simulink model "controller_AWBT"  (R2015a)
settings: Solver=ode5  StartTime=0.0  StopTime=9  FixedStep=1e-4  MaxStep=1e-3  RelTol=1e-3
values from neighbouring files (symbols this model uses):
  Ap = A    [main_matlab_observer.m]    (also in plant.mat = [-1.63570125246 -486.357845111 0 0 486.287213279 -1.89932026)
  Bp = B    [main_matlab_observer.m]    (also in plant.mat = [-8.88712865174  3.42023387272; 4.6056577442  -2.14780344563)
  Cp = C    [main_matlab_observer.m]    (also in plant.mat = [0.096809951598  0.0841099123333  0.0902904274622  -0.004558)
  Hp = E    [main_matlab_observer.m]    (also in plant.mat = [0.54311538907 1.14048132564 -4.51921348509 6.79727761668])
  Lambda = [-276.84208391  -85.2533778264; -2069.93210823  -868.288850378; 79.3180780662  -82.3979419554; -14381.7794783  -8216.05302909; -0.144673414091  -0.164940951057; 0.726371656625  -0.617647342535]    [controller_khat.mat]    (also in main_matlab_controller.m = X/M)
libraries: cstblocks x2, simulink x1
settings Model: Creator=p4wp4w  LastModifiedBy=p4wp4w
settings SolverCC: AlgebraicLoopSolver=LineSearch

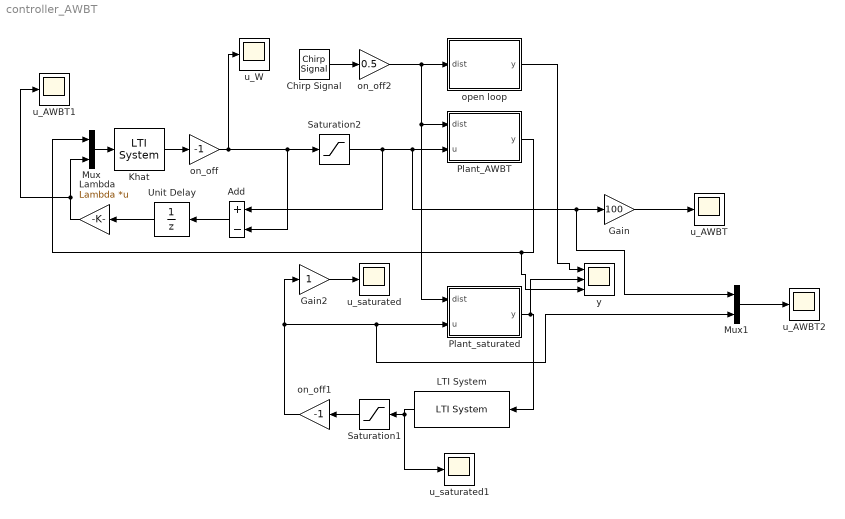
== system controller_AWBT ==
  Add : Sum  Inputs=+-
  Chirp Signal : simulink/Sources/Chirp Signal  f1=0.1  T=9  f2=90
  Gain : Gain  Gain=100
  Gain2 : Gain
  Khat : cstblocks/LTI System  sys=K_hat  IC=[]
  LTI System : cstblocks/LTI System  sys=controller_implemented  IC=[]
  Lambda : Gain  Gain=Lambda  Multiplication=Matrix(K*u)
  Mux : Mux  Inputs=2
  Mux1 : Mux  Inputs=2
  Plant_AWBT : Subsystem
  Plant_saturated : Subsystem
  Saturation1 : Saturate  UpperLimit=0.1  LowerLimit=-0.1
  Saturation2 : Saturate  UpperLimit=0.1  LowerLimit=-0.1
  Unit Delay : UnitDelay  SampleTime=-1
  on_off : Gain  Gain=-1
  on_off1 : Gain  Gain=-1
  on_off2 : Gain  Gain=0.5
  open loop : Subsystem
  u_AWBT : Scope
      settings: YMin=-0.75  YMax=0.75
  u_AWBT1 : Scope
      settings: YMin=-35  YMax=35  SaveName=ScopeData5
  u_AWBT2 : Scope
      settings: ShowLegends=on  YMin=-0.75  YMax=0.75  SaveName=ScopeData6
  u_W : Scope
      settings: YMin=-500  YMax=500  SaveName=ScopeData3
  u_saturated : Scope
      settings: YMin=47.5  YMax=52.5  SaveName=ScopeData2
  u_saturated1 : Scope
      settings: TimeRange=4.684200000000001  YMin=-0.5  YMax=0.45  SaveName=ScopeData4
  y : Scope  NumInputPorts=3
      settings: ShowLegends=on  YMin=-4~-5~-5  YMax=4~5~5
  wires:
  Mux/1 -> Khat/1
  Plant_AWBT/1(y) -> y/3, Mux/1
  Khat/1 -> on_off/1
  Plant_saturated/1(y) -> y/2, LTI System/1
  on_off1/1 -> Mux1/2, Plant_saturated/2(u), Gain2/1
  Lambda/1 -> u_AWBT1/1, Mux/2
  on_off/1 -> u_W/1, Add/2, Saturation2/1
  Saturation2/1 -> Add/1, Mux1/1, Gain/1, Plant_AWBT/2(u)
  Add/1 -> Unit Delay/1
  Gain/1 -> u_AWBT/1
  Gain2/1 -> u_saturated/1
  Unit Delay/1 -> Lambda/1
  on_off2/1 -> open loop/1(dist), Plant_saturated/1(dist), Plant_AWBT/1(dist)
  Chirp Signal/1 -> on_off2/1
  LTI System/1 -> Saturation1/1, u_saturated1/1
  open loop/1(y) -> y/1
  Saturation1/1 -> on_off1/1
  Mux1/1 -> u_AWBT2/1

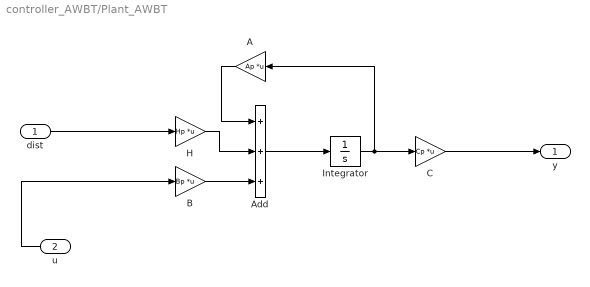
== system controller_AWBT/Plant_AWBT ==
  dist : Inport
  u : Inport  Port=2
  A : Gain  Gain=Ap  Multiplication=Matrix(K*u)
  Add : Sum  Inputs=+++
  B : Gain  Gain=Bp  Multiplication=Matrix(K*u)
  C : Gain  Gain=Cp  Multiplication=Matrix(K*u)
  H : Gain  Gain=Hp  Multiplication=Matrix(K*u)
  Integrator : Integrator
  y : Outport
  wires:
  Add/1 -> Integrator/1
  H/1 -> Add/2
  A/1 -> Add/1
  dist/1 -> H/1
  B/1 -> Add/3
  Integrator/1 -> C/1, A/1
  u/1 -> B/1
  C/1 -> y/1

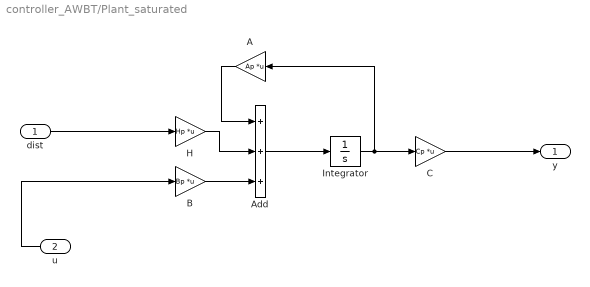
== system controller_AWBT/Plant_saturated ==
  dist : Inport
  u : Inport  Port=2
  A : Gain  Gain=Ap  Multiplication=Matrix(K*u)
  Add : Sum  Inputs=+++
  B : Gain  Gain=Bp  Multiplication=Matrix(K*u)
  C : Gain  Gain=Cp  Multiplication=Matrix(K*u)
  H : Gain  Gain=Hp  Multiplication=Matrix(K*u)
  Integrator : Integrator
  y : Outport
  wires:
  u/1 -> B/1
  Integrator/1 -> A/1, C/1
  B/1 -> Add/3
  dist/1 -> H/1
  A/1 -> Add/1
  H/1 -> Add/2
  Add/1 -> Integrator/1
  C/1 -> y/1

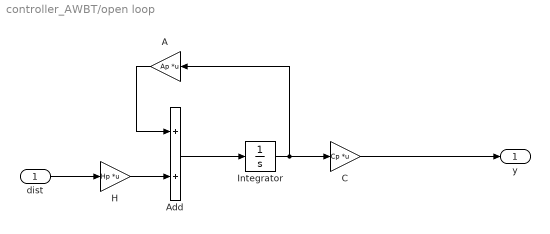
== system controller_AWBT/open loop ==
  dist : Inport
  A : Gain  Gain=Ap  Multiplication=Matrix(K*u)
  Add : Sum
  C : Gain  Gain=Cp  Multiplication=Matrix(K*u)
  H : Gain  Gain=Hp  Multiplication=Matrix(K*u)
  Integrator : Integrator
  y : Outport
  wires:
  Integrator/1 -> A/1, C/1
  dist/1 -> H/1
  A/1 -> Add/1
  H/1 -> Add/2
  Add/1 -> Integrator/1
  C/1 -> y/1
